simulink model "CPDemo"  (Simulink 7.8)
settings: Solver=ode1  StartTime=0  StopTime=250  FixedStep=1  RelTol=1e-3
libraries: DRRALibrary x105, simulink x10
settings Model: Creator=Administrator  LastModifiedBy=shuol
settings SolverCC: AlgebraicLoopSolver=LineSearch
settings OptimizationCC: BlockReduction=off  BooleanDataType=off  ConditionallyExecuteInputs=off

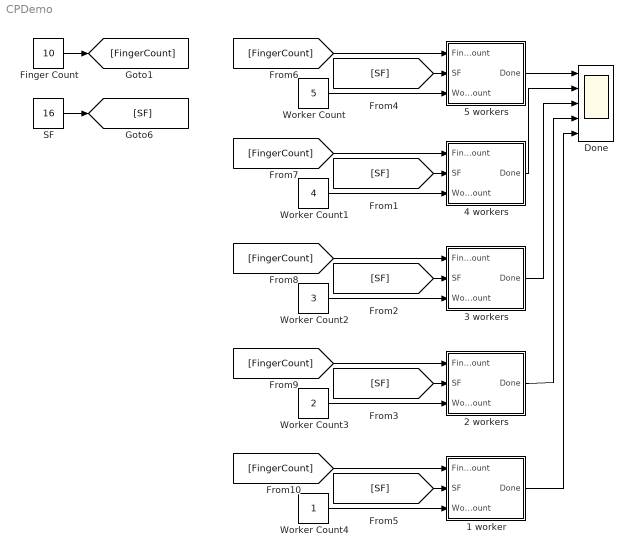
== system CPDemo ==
  1 worker : Subsystem
  2 workers : Subsystem
  3 workers : Subsystem
  4 workers : Subsystem
  5 workers : Subsystem
  Done : Scope  NumInputPorts=5
      settings: TickLabels=on  YMin=-1~-1~-1~-1~-1  YMax=2~2~2~2~2
  Finger Count : Constant  Value=10  SampleTime=1
  SF : Constant  Value=16  SampleTime=1
  Worker Count : Constant  Value=5  SampleTime=1
  Worker Count1 : Constant  Value=4  SampleTime=1
  Worker Count2 : Constant  Value=3  SampleTime=1
  Worker Count3 : Constant  Value=2  SampleTime=1
  Worker Count4 : Constant  SampleTime=1
  wires:
  [SF] -> 5 workers/2(SF)
  Worker Count/1 -> 5 workers/3(Worker Count)
  5 workers/1(Done) -> Done/1
  [SF] -> 4 workers/2(SF)
  Worker Count1/1 -> 4 workers/3(Worker Count)
  [SF] -> 3 workers/2(SF)
  Worker Count2/1 -> 3 workers/3(Worker Count)
  [SF] -> 2 workers/2(SF)
  Worker Count3/1 -> 2 workers/3(Worker Count)
  [SF] -> 1 worker/2(SF)
  Worker Count4/1 -> 1 worker/3(Worker Count)
  4 workers/1(Done) -> Done/2
  3 workers/1(Done) -> Done/3
  2 workers/1(Done) -> Done/4
  1 worker/1(Done) -> Done/5
  SF/1 -> [SF]
  Finger Count/1 -> [FingerCount]
  [FingerCount] -> 5 workers/1(Finger Count)
  [FingerCount] -> 1 worker/1(Finger Count)
  [FingerCount] -> 2 workers/1(Finger Count)
  [FingerCount] -> 3 workers/1(Finger Count)
  [FingerCount] -> 4 workers/1(Finger Count)

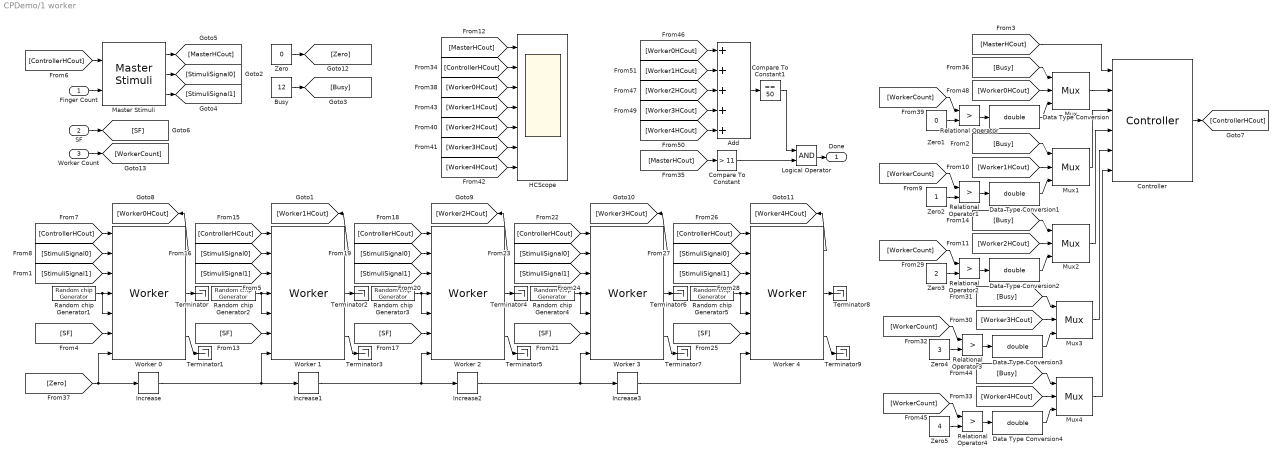
== system CPDemo/1 worker ==
  Finger Count : Inport
  SF : Inport  Port=2
  Worker Count : Inport  Port=3
  Add : Sum  Inputs=+++++  SampleTime=1
  Busy : Constant  Value=12  SampleTime=1
  Compare To Constant : simulink/Logic and Bit Operations/Compare To Constant  relop=>  const=11  OutDataTypeStr=uint8
  Compare To Constant1 : simulink/Logic and Bit Operations/Compare To Constant  relop===  const=50  OutDataTypeStr=uint8
  Controller : DRRALibrary/Function Library/Correlation Pool/Used Functions/Extended Functions/Controller
  Data Type Conversion{,1..4} (5 alike) : DataTypeConversion  OutDataTypeStr=double
  HCScope : Scope  NumInputPorts=7
      settings: TickLabels=on  YMin=-1~-1~-1~-1~-1~-1~-1  YMax=16~16~16~16~16~16~16
  Increase{,1..3} (4 alike) : DRRALibrary/Simulation Functions/Base Functions/Increase  SystemSampleTime=-1
  Logical Operator : Logic  AllPortsSameDT=off  OutDataTypeStr=boolean
  Master Stimuli : DRRALibrary/Function Library/Correlation Pool/Used Functions/Extended Functions/Master Stimuli
  Mux{,1..4} (5 alike) : DRRALibrary/Simulation Functions/Base Functions/Mux
  Random chip Generator{1..5} (5 alike) : DRRALibrary/Function Library/Correlation Pool/Used Functions/Extended Functions/Random chip Generator
  Relational Operator{,1..4} (5 alike) : RelationalOperator  Operator=>  OutDataTypeStr=boolean
  Terminator{,1..9} (10 alike) : Terminator
  Worker {0..4} (5 alike) : DRRALibrary/Function Library/Correlation Pool/Used Functions/Extended Functions/Worker 
  Zero : Constant  Value=0  SampleTime=1
  Zero1 : Constant  Value=0  SampleTime=1
  Zero2 : Constant  SampleTime=1
  Zero3 : Constant  Value=2  SampleTime=1
  Zero4 : Constant  Value=3  SampleTime=1
  Zero5 : Constant  Value=4  SampleTime=1
  Done : Outport
  wires:
  Data Type Conversion/1 -> Mux/3
  Relational Operator/1 -> Data Type Conversion/1
  Worker Count/1 -> [WorkerCount]
  [Zero] -> Worker 0/7, Increase/1
  Zero/1 -> [Zero]
  Busy/1 -> [Busy]
  Finger Count/1 -> Master Stimuli/2
  Worker 4/3 -> Terminator9/1
  Worker 4/2 -> Terminator8/1
  Worker 3/2 -> Terminator6/1
  Worker 3/3 -> Terminator7/1
  Worker 2/3 -> Terminator5/1
  Worker 2/2 -> Terminator4/1
  Worker 1/3 -> Terminator3/1
  Worker 1/2 -> Terminator2/1
  Worker 0/3 -> Terminator1/1
  Worker 0/2 -> Terminator/1
  SF/1 -> [SF]
  Master Stimuli/3 -> [StimuliSignal1]
  Worker 4/1 -> [Worker4HCout]
  Increase3/1 -> Worker 4/7
  [SF] -> Worker 4/6
  [StimuliSignal1] -> Worker 4/3
  Random chip Generator5/1 -> Worker 4/4, Worker 4/5
  [StimuliSignal0] -> Worker 4/2
  [ControllerHCout] -> Worker 4/1
  Worker 3/1 -> [Worker3HCout]
  Increase2/1 -> Worker 3/7, Increase3/1
  [SF] -> Worker 3/6
  [StimuliSignal1] -> Worker 3/3
  Random chip Generator4/1 -> Worker 3/5, Worker 3/4
  [StimuliSignal0] -> Worker 3/2
  [ControllerHCout] -> Worker 3/1
  Worker 2/1 -> [Worker2HCout]
  Increase1/1 -> Increase2/1, Worker 2/7
  [SF] -> Worker 2/6
  [StimuliSignal1] -> Worker 2/3
  Random chip Generator3/1 -> Worker 2/4, Worker 2/5
  [StimuliSignal0] -> Worker 2/2
  [ControllerHCout] -> Worker 2/1
  Worker 1/1 -> [Worker1HCout]
  Increase/1 -> Worker 1/7, Increase1/1
  [SF] -> Worker 1/6
  [StimuliSignal1] -> Worker 1/3
  Random chip Generator2/1 -> Worker 1/5, Worker 1/4
  [StimuliSignal0] -> Worker 1/2
  [ControllerHCout] -> Worker 1/1
  Worker 0/1 -> [Worker0HCout]
  [SF] -> Worker 0/6
  [StimuliSignal1] -> Worker 0/3
  [ControllerHCout] -> Master Stimuli/1
  Random chip Generator1/1 -> Worker 0/4, Worker 0/5
  [StimuliSignal0] -> Worker 0/2
  [ControllerHCout] -> Worker 0/1
  [MasterHCout] -> Controller/1
  Controller/1 -> [ControllerHCout]
  Master Stimuli/2 -> [StimuliSignal0]
  Master Stimuli/1 -> [MasterHCout]
  [MasterHCout] -> Compare To Constant/1
  [MasterHCout] -> HCScope/1
  [ControllerHCout] -> HCScope/2
  [Worker0HCout] -> Mux/2
  [WorkerCount] -> Relational Operator/1
  Zero1/1 -> Relational Operator/2
  [Worker4HCout] -> HCScope/7
  [Worker3HCout] -> HCScope/6
  [Worker2HCout] -> HCScope/5
  [Worker1HCout] -> HCScope/4
  [Worker0HCout] -> HCScope/3
  [Busy] -> Mux/1
  Data Type Conversion1/1 -> Mux1/3
  Relational Operator1/1 -> Data Type Conversion1/1
  [Worker1HCout] -> Mux1/2
  [WorkerCount] -> Relational Operator1/1
  Zero2/1 -> Relational Operator1/2
  [Busy] -> Mux1/1
  Data Type Conversion2/1 -> Mux2/3
  Relational Operator2/1 -> Data Type Conversion2/1
  [Worker2HCout] -> Mux2/2
  [WorkerCount] -> Relational Operator2/1
  Zero3/1 -> Relational Operator2/2
  [Busy] -> Mux2/1
  Data Type Conversion3/1 -> Mux3/3
  Relational Operator3/1 -> Data Type Conversion3/1
  [Worker3HCout] -> Mux3/2
  [WorkerCount] -> Relational Operator3/1
  Zero4/1 -> Relational Operator3/2
  [Busy] -> Mux3/1
  Data Type Conversion4/1 -> Mux4/3
  Relational Operator4/1 -> Data Type Conversion4/1
  [Worker4HCout] -> Mux4/2
  [WorkerCount] -> Relational Operator4/1
  Zero5/1 -> Relational Operator4/2
  [Busy] -> Mux4/1
  Mux/1 -> Controller/2
  Mux1/1 -> Controller/3
  Mux2/1 -> Controller/4
  Mux3/1 -> Controller/5
  Mux4/1 -> Controller/6
  [Worker0HCout] -> Add/1
  [Worker1HCout] -> Add/2
  [Worker2HCout] -> Add/3
  [Worker3HCout] -> Add/4
  [Worker4HCout] -> Add/5
  Add/1 -> Compare To Constant1/1
  Compare To Constant/1 -> Logical Operator/2
  Compare To Constant1/1 -> Logical Operator/1
  Logical Operator/1 -> Done/1

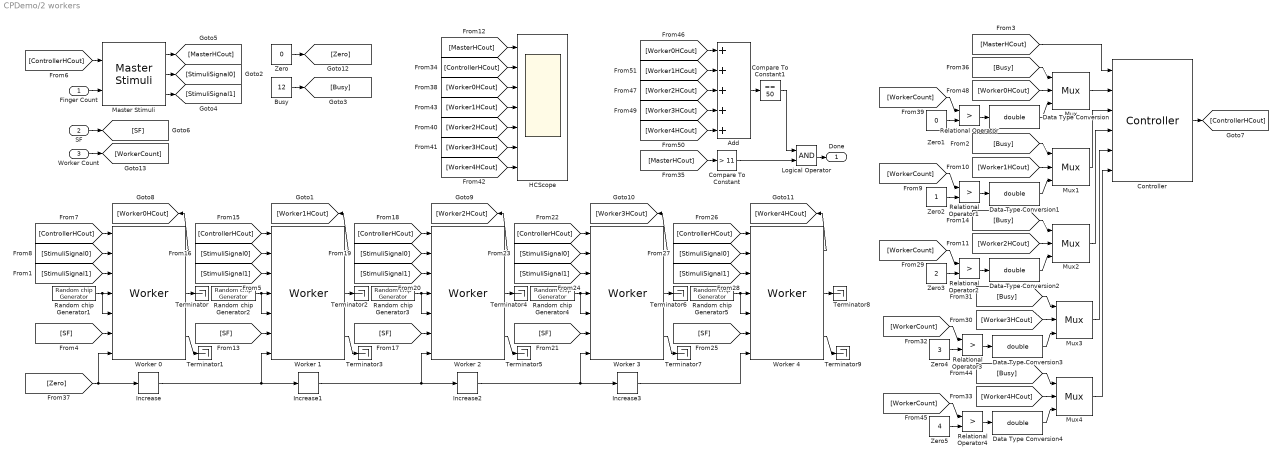
== system CPDemo/2 workers ==
  Finger Count : Inport
  SF : Inport  Port=2
  Worker Count : Inport  Port=3
  Add : Sum  Inputs=+++++  SampleTime=1
  Busy : Constant  Value=12  SampleTime=1
  Compare To Constant : simulink/Logic and Bit Operations/Compare To Constant  relop=>  const=11  OutDataTypeStr=uint8
  Compare To Constant1 : simulink/Logic and Bit Operations/Compare To Constant  relop===  const=50  OutDataTypeStr=uint8
  Controller : DRRALibrary/Function Library/Correlation Pool/Used Functions/Extended Functions/Controller
  Data Type Conversion{,1..4} (5 alike) : DataTypeConversion  OutDataTypeStr=double
  HCScope : Scope  NumInputPorts=7
      settings: TickLabels=on  YMin=-1~-1~-1~-1~-1~-1~-1  YMax=16~16~16~16~16~16~16
  Increase{,1..3} (4 alike) : DRRALibrary/Simulation Functions/Base Functions/Increase  SystemSampleTime=-1
  Logical Operator : Logic  AllPortsSameDT=off  OutDataTypeStr=boolean
  Master Stimuli : DRRALibrary/Function Library/Correlation Pool/Used Functions/Extended Functions/Master Stimuli
  Mux{,1..4} (5 alike) : DRRALibrary/Simulation Functions/Base Functions/Mux
  Random chip Generator{1..5} (5 alike) : DRRALibrary/Function Library/Correlation Pool/Used Functions/Extended Functions/Random chip Generator
  Relational Operator{,1..4} (5 alike) : RelationalOperator  Operator=>  OutDataTypeStr=boolean
  Terminator{,1..9} (10 alike) : Terminator
  Worker {0..4} (5 alike) : DRRALibrary/Function Library/Correlation Pool/Used Functions/Extended Functions/Worker 
  Zero : Constant  Value=0  SampleTime=1
  Zero1 : Constant  Value=0  SampleTime=1
  Zero2 : Constant  SampleTime=1
  Zero3 : Constant  Value=2  SampleTime=1
  Zero4 : Constant  Value=3  SampleTime=1
  Zero5 : Constant  Value=4  SampleTime=1
  Done : Outport
  wires:
  Logical Operator/1 -> Done/1
  Compare To Constant1/1 -> Logical Operator/1
  Compare To Constant/1 -> Logical Operator/2
  Add/1 -> Compare To Constant1/1
  [Worker4HCout] -> Add/5
  [Worker3HCout] -> Add/4
  [Worker2HCout] -> Add/3
  [Worker1HCout] -> Add/2
  [Worker0HCout] -> Add/1
  Mux4/1 -> Controller/6
  Mux3/1 -> Controller/5
  Mux2/1 -> Controller/4
  Mux1/1 -> Controller/3
  Mux/1 -> Controller/2
  [Busy] -> Mux4/1
  Zero5/1 -> Relational Operator4/2
  [WorkerCount] -> Relational Operator4/1
  [Worker4HCout] -> Mux4/2
  Relational Operator4/1 -> Data Type Conversion4/1
  Data Type Conversion4/1 -> Mux4/3
  [Busy] -> Mux3/1
  Zero4/1 -> Relational Operator3/2
  [WorkerCount] -> Relational Operator3/1
  [Worker3HCout] -> Mux3/2
  Relational Operator3/1 -> Data Type Conversion3/1
  Data Type Conversion3/1 -> Mux3/3
  [Busy] -> Mux2/1
  Zero3/1 -> Relational Operator2/2
  [WorkerCount] -> Relational Operator2/1
  [Worker2HCout] -> Mux2/2
  Relational Operator2/1 -> Data Type Conversion2/1
  Data Type Conversion2/1 -> Mux2/3
  [Busy] -> Mux1/1
  Zero2/1 -> Relational Operator1/2
  [WorkerCount] -> Relational Operator1/1
  [Worker1HCout] -> Mux1/2
  Relational Operator1/1 -> Data Type Conversion1/1
  Data Type Conversion1/1 -> Mux1/3
  [Busy] -> Mux/1
  [Worker0HCout] -> HCScope/3
  [Worker1HCout] -> HCScope/4
  [Worker2HCout] -> HCScope/5
  [Worker3HCout] -> HCScope/6
  [Worker4HCout] -> HCScope/7
  Zero1/1 -> Relational Operator/2
  [WorkerCount] -> Relational Operator/1
  [Worker0HCout] -> Mux/2
  [ControllerHCout] -> HCScope/2
  [MasterHCout] -> HCScope/1
  [MasterHCout] -> Compare To Constant/1
  Master Stimuli/1 -> [MasterHCout]
  Master Stimuli/2 -> [StimuliSignal0]
  Controller/1 -> [ControllerHCout]
  [MasterHCout] -> Controller/1
  [ControllerHCout] -> Worker 0/1
  [StimuliSignal0] -> Worker 0/2
  Random chip Generator1/1 -> Worker 0/5, Worker 0/4
  [ControllerHCout] -> Master Stimuli/1
  [StimuliSignal1] -> Worker 0/3
  [SF] -> Worker 0/6
  Worker 0/1 -> [Worker0HCout]
  [ControllerHCout] -> Worker 1/1
  [StimuliSignal0] -> Worker 1/2
  Random chip Generator2/1 -> Worker 1/4, Worker 1/5
  [StimuliSignal1] -> Worker 1/3
  [SF] -> Worker 1/6
  Increase/1 -> Increase1/1, Worker 1/7
  Worker 1/1 -> [Worker1HCout]
  [ControllerHCout] -> Worker 2/1
  [StimuliSignal0] -> Worker 2/2
  Random chip Generator3/1 -> Worker 2/5, Worker 2/4
  [StimuliSignal1] -> Worker 2/3
  [SF] -> Worker 2/6
  Increase1/1 -> Worker 2/7, Increase2/1
  Worker 2/1 -> [Worker2HCout]
  [ControllerHCout] -> Worker 3/1
  [StimuliSignal0] -> Worker 3/2
  Random chip Generator4/1 -> Worker 3/4, Worker 3/5
  [StimuliSignal1] -> Worker 3/3
  [SF] -> Worker 3/6
  Increase2/1 -> Increase3/1, Worker 3/7
  Worker 3/1 -> [Worker3HCout]
  [ControllerHCout] -> Worker 4/1
  [StimuliSignal0] -> Worker 4/2
  Random chip Generator5/1 -> Worker 4/5, Worker 4/4
  [StimuliSignal1] -> Worker 4/3
  [SF] -> Worker 4/6
  Increase3/1 -> Worker 4/7
  Worker 4/1 -> [Worker4HCout]
  Master Stimuli/3 -> [StimuliSignal1]
  SF/1 -> [SF]
  Worker 0/2 -> Terminator/1
  Worker 0/3 -> Terminator1/1
  Worker 1/2 -> Terminator2/1
  Worker 1/3 -> Terminator3/1
  Worker 2/2 -> Terminator4/1
  Worker 2/3 -> Terminator5/1
  Worker 3/3 -> Terminator7/1
  Worker 3/2 -> Terminator6/1
  Worker 4/2 -> Terminator8/1
  Worker 4/3 -> Terminator9/1
  Finger Count/1 -> Master Stimuli/2
  Busy/1 -> [Busy]
  Zero/1 -> [Zero]
  [Zero] -> Increase/1, Worker 0/7
  Worker Count/1 -> [WorkerCount]
  Relational Operator/1 -> Data Type Conversion/1
  Data Type Conversion/1 -> Mux/3

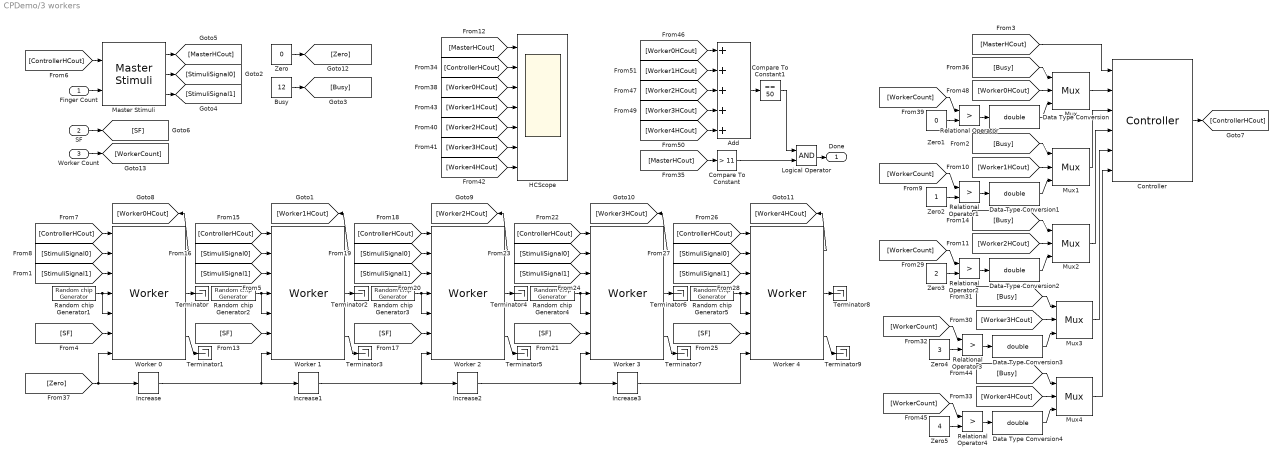
== system CPDemo/3 workers ==
  Finger Count : Inport
  SF : Inport  Port=2
  Worker Count : Inport  Port=3
  Add : Sum  Inputs=+++++  SampleTime=1
  Busy : Constant  Value=12  SampleTime=1
  Compare To Constant : simulink/Logic and Bit Operations/Compare To Constant  relop=>  const=11  OutDataTypeStr=uint8
  Compare To Constant1 : simulink/Logic and Bit Operations/Compare To Constant  relop===  const=50  OutDataTypeStr=uint8
  Controller : DRRALibrary/Function Library/Correlation Pool/Used Functions/Extended Functions/Controller
  Data Type Conversion{,1..4} (5 alike) : DataTypeConversion  OutDataTypeStr=double
  HCScope : Scope  NumInputPorts=7
      settings: TickLabels=on  YMin=-1~-1~-1~-1~-1~-1~-1  YMax=16~16~16~16~16~16~16
  Increase{,1..3} (4 alike) : DRRALibrary/Simulation Functions/Base Functions/Increase  SystemSampleTime=-1
  Logical Operator : Logic  AllPortsSameDT=off  OutDataTypeStr=boolean
  Master Stimuli : DRRALibrary/Function Library/Correlation Pool/Used Functions/Extended Functions/Master Stimuli
  Mux{,1..4} (5 alike) : DRRALibrary/Simulation Functions/Base Functions/Mux
  Random chip Generator{1..5} (5 alike) : DRRALibrary/Function Library/Correlation Pool/Used Functions/Extended Functions/Random chip Generator
  Relational Operator{,1..4} (5 alike) : RelationalOperator  Operator=>  OutDataTypeStr=boolean
  Terminator{,1..9} (10 alike) : Terminator
  Worker {0..4} (5 alike) : DRRALibrary/Function Library/Correlation Pool/Used Functions/Extended Functions/Worker 
  Zero : Constant  Value=0  SampleTime=1
  Zero1 : Constant  Value=0  SampleTime=1
  Zero2 : Constant  SampleTime=1
  Zero3 : Constant  Value=2  SampleTime=1
  Zero4 : Constant  Value=3  SampleTime=1
  Zero5 : Constant  Value=4  SampleTime=1
  Done : Outport
  wires:
  Data Type Conversion/1 -> Mux/3
  Relational Operator/1 -> Data Type Conversion/1
  Worker Count/1 -> [WorkerCount]
  [Zero] -> Worker 0/7, Increase/1
  Zero/1 -> [Zero]
  Busy/1 -> [Busy]
  Finger Count/1 -> Master Stimuli/2
  Worker 4/3 -> Terminator9/1
  Worker 4/2 -> Terminator8/1
  Worker 3/2 -> Terminator6/1
  Worker 3/3 -> Terminator7/1
  Worker 2/3 -> Terminator5/1
  Worker 2/2 -> Terminator4/1
  Worker 1/3 -> Terminator3/1
  Worker 1/2 -> Terminator2/1
  Worker 0/3 -> Terminator1/1
  Worker 0/2 -> Terminator/1
  SF/1 -> [SF]
  Master Stimuli/3 -> [StimuliSignal1]
  Worker 4/1 -> [Worker4HCout]
  Increase3/1 -> Worker 4/7
  [SF] -> Worker 4/6
  [StimuliSignal1] -> Worker 4/3
  Random chip Generator5/1 -> Worker 4/4, Worker 4/5
  [StimuliSignal0] -> Worker 4/2
  [ControllerHCout] -> Worker 4/1
  Worker 3/1 -> [Worker3HCout]
  Increase2/1 -> Worker 3/7, Increase3/1
  [SF] -> Worker 3/6
  [StimuliSignal1] -> Worker 3/3
  Random chip Generator4/1 -> Worker 3/5, Worker 3/4
  [StimuliSignal0] -> Worker 3/2
  [ControllerHCout] -> Worker 3/1
  Worker 2/1 -> [Worker2HCout]
  Increase1/1 -> Increase2/1, Worker 2/7
  [SF] -> Worker 2/6
  [StimuliSignal1] -> Worker 2/3
  Random chip Generator3/1 -> Worker 2/4, Worker 2/5
  [StimuliSignal0] -> Worker 2/2
  [ControllerHCout] -> Worker 2/1
  Worker 1/1 -> [Worker1HCout]
  Increase/1 -> Worker 1/7, Increase1/1
  [SF] -> Worker 1/6
  [StimuliSignal1] -> Worker 1/3
  Random chip Generator2/1 -> Worker 1/5, Worker 1/4
  [StimuliSignal0] -> Worker 1/2
  [ControllerHCout] -> Worker 1/1
  Worker 0/1 -> [Worker0HCout]
  [SF] -> Worker 0/6
  [StimuliSignal1] -> Worker 0/3
  [ControllerHCout] -> Master Stimuli/1
  Random chip Generator1/1 -> Worker 0/4, Worker 0/5
  [StimuliSignal0] -> Worker 0/2
  [ControllerHCout] -> Worker 0/1
  [MasterHCout] -> Controller/1
  Controller/1 -> [ControllerHCout]
  Master Stimuli/2 -> [StimuliSignal0]
  Master Stimuli/1 -> [MasterHCout]
  [MasterHCout] -> Compare To Constant/1
  [MasterHCout] -> HCScope/1
  [ControllerHCout] -> HCScope/2
  [Worker0HCout] -> Mux/2
  [WorkerCount] -> Relational Operator/1
  Zero1/1 -> Relational Operator/2
  [Worker4HCout] -> HCScope/7
  [Worker3HCout] -> HCScope/6
  [Worker2HCout] -> HCScope/5
  [Worker1HCout] -> HCScope/4
  [Worker0HCout] -> HCScope/3
  [Busy] -> Mux/1
  Data Type Conversion1/1 -> Mux1/3
  Relational Operator1/1 -> Data Type Conversion1/1
  [Worker1HCout] -> Mux1/2
  [WorkerCount] -> Relational Operator1/1
  Zero2/1 -> Relational Operator1/2
  [Busy] -> Mux1/1
  Data Type Conversion2/1 -> Mux2/3
  Relational Operator2/1 -> Data Type Conversion2/1
  [Worker2HCout] -> Mux2/2
  [WorkerCount] -> Relational Operator2/1
  Zero3/1 -> Relational Operator2/2
  [Busy] -> Mux2/1
  Data Type Conversion3/1 -> Mux3/3
  Relational Operator3/1 -> Data Type Conversion3/1
  [Worker3HCout] -> Mux3/2
  [WorkerCount] -> Relational Operator3/1
  Zero4/1 -> Relational Operator3/2
  [Busy] -> Mux3/1
  Data Type Conversion4/1 -> Mux4/3
  Relational Operator4/1 -> Data Type Conversion4/1
  [Worker4HCout] -> Mux4/2
  [WorkerCount] -> Relational Operator4/1
  Zero5/1 -> Relational Operator4/2
  [Busy] -> Mux4/1
  Mux/1 -> Controller/2
  Mux1/1 -> Controller/3
  Mux2/1 -> Controller/4
  Mux3/1 -> Controller/5
  Mux4/1 -> Controller/6
  [Worker0HCout] -> Add/1
  [Worker1HCout] -> Add/2
  [Worker2HCout] -> Add/3
  [Worker3HCout] -> Add/4
  [Worker4HCout] -> Add/5
  Add/1 -> Compare To Constant1/1
  Compare To Constant/1 -> Logical Operator/2
  Compare To Constant1/1 -> Logical Operator/1
  Logical Operator/1 -> Done/1

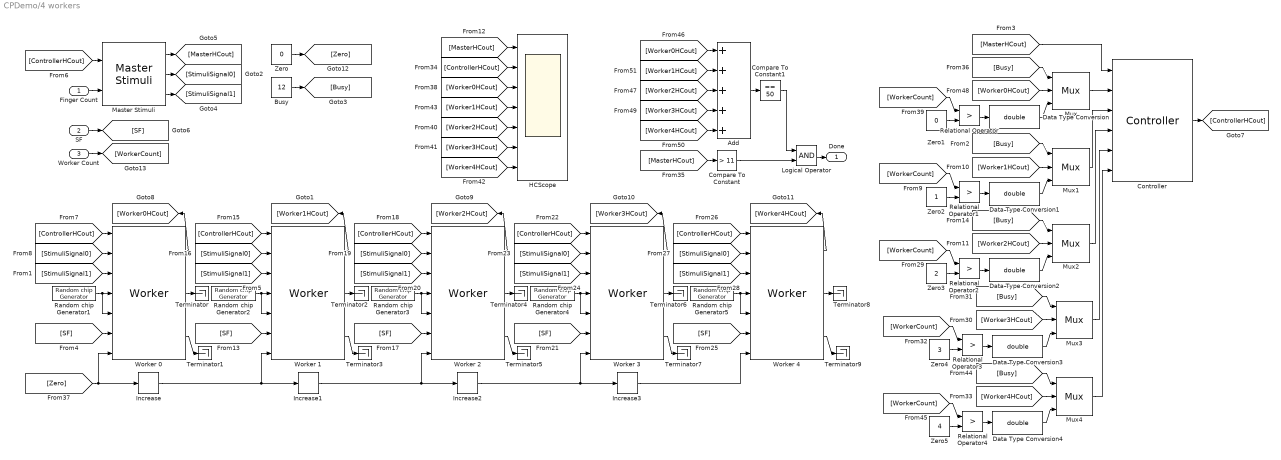
== system CPDemo/4 workers ==
  Finger Count : Inport
  SF : Inport  Port=2
  Worker Count : Inport  Port=3
  Add : Sum  Inputs=+++++  SampleTime=1
  Busy : Constant  Value=12  SampleTime=1
  Compare To Constant : simulink/Logic and Bit Operations/Compare To Constant  relop=>  const=11  OutDataTypeStr=uint8
  Compare To Constant1 : simulink/Logic and Bit Operations/Compare To Constant  relop===  const=50  OutDataTypeStr=uint8
  Controller : DRRALibrary/Function Library/Correlation Pool/Used Functions/Extended Functions/Controller
  Data Type Conversion{,1..4} (5 alike) : DataTypeConversion  OutDataTypeStr=double
  HCScope : Scope  NumInputPorts=7
      settings: TickLabels=on  YMin=-1~-1~-1~-1~-1~-1~-1  YMax=16~16~16~16~16~16~16
  Increase{,1..3} (4 alike) : DRRALibrary/Simulation Functions/Base Functions/Increase  SystemSampleTime=-1
  Logical Operator : Logic  AllPortsSameDT=off  OutDataTypeStr=boolean
  Master Stimuli : DRRALibrary/Function Library/Correlation Pool/Used Functions/Extended Functions/Master Stimuli
  Mux{,1..4} (5 alike) : DRRALibrary/Simulation Functions/Base Functions/Mux
  Random chip Generator{1..5} (5 alike) : DRRALibrary/Function Library/Correlation Pool/Used Functions/Extended Functions/Random chip Generator
  Relational Operator{,1..4} (5 alike) : RelationalOperator  Operator=>  OutDataTypeStr=boolean
  Terminator{,1..9} (10 alike) : Terminator
  Worker {0..4} (5 alike) : DRRALibrary/Function Library/Correlation Pool/Used Functions/Extended Functions/Worker 
  Zero : Constant  Value=0  SampleTime=1
  Zero1 : Constant  Value=0  SampleTime=1
  Zero2 : Constant  SampleTime=1
  Zero3 : Constant  Value=2  SampleTime=1
  Zero4 : Constant  Value=3  SampleTime=1
  Zero5 : Constant  Value=4  SampleTime=1
  Done : Outport
  wires:
  Logical Operator/1 -> Done/1
  Compare To Constant1/1 -> Logical Operator/1
  Compare To Constant/1 -> Logical Operator/2
  Add/1 -> Compare To Constant1/1
  [Worker4HCout] -> Add/5
  [Worker3HCout] -> Add/4
  [Worker2HCout] -> Add/3
  [Worker1HCout] -> Add/2
  [Worker0HCout] -> Add/1
  Mux4/1 -> Controller/6
  Mux3/1 -> Controller/5
  Mux2/1 -> Controller/4
  Mux1/1 -> Controller/3
  Mux/1 -> Controller/2
  [Busy] -> Mux4/1
  Zero5/1 -> Relational Operator4/2
  [WorkerCount] -> Relational Operator4/1
  [Worker4HCout] -> Mux4/2
  Relational Operator4/1 -> Data Type Conversion4/1
  Data Type Conversion4/1 -> Mux4/3
  [Busy] -> Mux3/1
  Zero4/1 -> Relational Operator3/2
  [WorkerCount] -> Relational Operator3/1
  [Worker3HCout] -> Mux3/2
  Relational Operator3/1 -> Data Type Conversion3/1
  Data Type Conversion3/1 -> Mux3/3
  [Busy] -> Mux2/1
  Zero3/1 -> Relational Operator2/2
  [WorkerCount] -> Relational Operator2/1
  [Worker2HCout] -> Mux2/2
  Relational Operator2/1 -> Data Type Conversion2/1
  Data Type Conversion2/1 -> Mux2/3
  [Busy] -> Mux1/1
  Zero2/1 -> Relational Operator1/2
  [WorkerCount] -> Relational Operator1/1
  [Worker1HCout] -> Mux1/2
  Relational Operator1/1 -> Data Type Conversion1/1
  Data Type Conversion1/1 -> Mux1/3
  [Busy] -> Mux/1
  [Worker0HCout] -> HCScope/3
  [Worker1HCout] -> HCScope/4
  [Worker2HCout] -> HCScope/5
  [Worker3HCout] -> HCScope/6
  [Worker4HCout] -> HCScope/7
  Zero1/1 -> Relational Operator/2
  [WorkerCount] -> Relational Operator/1
  [Worker0HCout] -> Mux/2
  [ControllerHCout] -> HCScope/2
  [MasterHCout] -> HCScope/1
  [MasterHCout] -> Compare To Constant/1
  Master Stimuli/1 -> [MasterHCout]
  Master Stimuli/2 -> [StimuliSignal0]
  Controller/1 -> [ControllerHCout]
  [MasterHCout] -> Controller/1
  [ControllerHCout] -> Worker 0/1
  [StimuliSignal0] -> Worker 0/2
  Random chip Generator1/1 -> Worker 0/5, Worker 0/4
  [ControllerHCout] -> Master Stimuli/1
  [StimuliSignal1] -> Worker 0/3
  [SF] -> Worker 0/6
  Worker 0/1 -> [Worker0HCout]
  [ControllerHCout] -> Worker 1/1
  [StimuliSignal0] -> Worker 1/2
  Random chip Generator2/1 -> Worker 1/4, Worker 1/5
  [StimuliSignal1] -> Worker 1/3
  [SF] -> Worker 1/6
  Increase/1 -> Increase1/1, Worker 1/7
  Worker 1/1 -> [Worker1HCout]
  [ControllerHCout] -> Worker 2/1
  [StimuliSignal0] -> Worker 2/2
  Random chip Generator3/1 -> Worker 2/5, Worker 2/4
  [StimuliSignal1] -> Worker 2/3
  [SF] -> Worker 2/6
  Increase1/1 -> Worker 2/7, Increase2/1
  Worker 2/1 -> [Worker2HCout]
  [ControllerHCout] -> Worker 3/1
  [StimuliSignal0] -> Worker 3/2
  Random chip Generator4/1 -> Worker 3/4, Worker 3/5
  [StimuliSignal1] -> Worker 3/3
  [SF] -> Worker 3/6
  Increase2/1 -> Increase3/1, Worker 3/7
  Worker 3/1 -> [Worker3HCout]
  [ControllerHCout] -> Worker 4/1
  [StimuliSignal0] -> Worker 4/2
  Random chip Generator5/1 -> Worker 4/5, Worker 4/4
  [StimuliSignal1] -> Worker 4/3
  [SF] -> Worker 4/6
  Increase3/1 -> Worker 4/7
  Worker 4/1 -> [Worker4HCout]
  Master Stimuli/3 -> [StimuliSignal1]
  SF/1 -> [SF]
  Worker 0/2 -> Terminator/1
  Worker 0/3 -> Terminator1/1
  Worker 1/2 -> Terminator2/1
  Worker 1/3 -> Terminator3/1
  Worker 2/2 -> Terminator4/1
  Worker 2/3 -> Terminator5/1
  Worker 3/3 -> Terminator7/1
  Worker 3/2 -> Terminator6/1
  Worker 4/2 -> Terminator8/1
  Worker 4/3 -> Terminator9/1
  Finger Count/1 -> Master Stimuli/2
  Busy/1 -> [Busy]
  Zero/1 -> [Zero]
  [Zero] -> Increase/1, Worker 0/7
  Worker Count/1 -> [WorkerCount]
  Relational Operator/1 -> Data Type Conversion/1
  Data Type Conversion/1 -> Mux/3

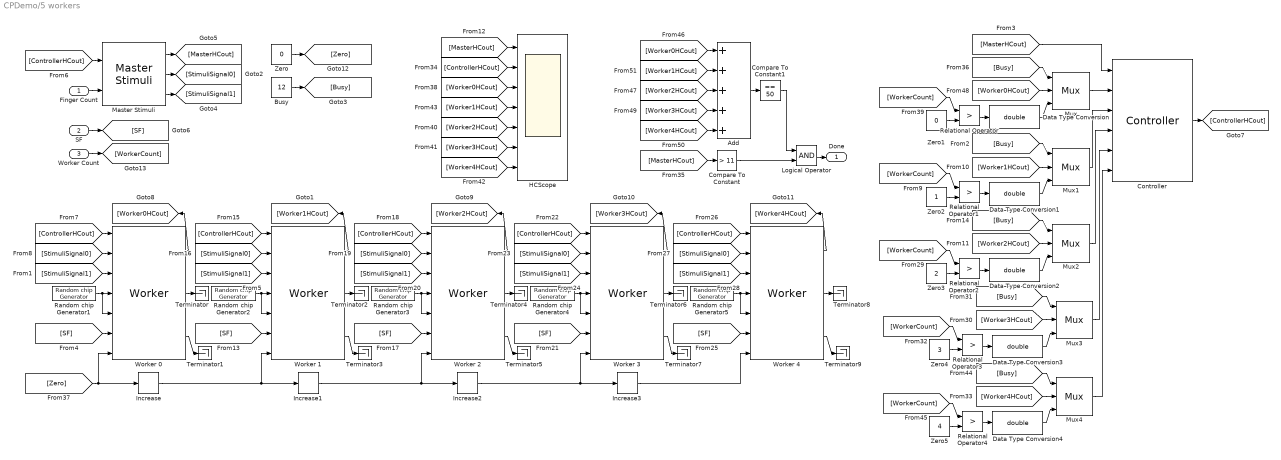
== system CPDemo/5 workers ==
  Finger Count : Inport
  SF : Inport  Port=2
  Worker Count : Inport  Port=3
  Add : Sum  Inputs=+++++  SampleTime=1
  Busy : Constant  Value=12  SampleTime=1
  Compare To Constant : simulink/Logic and Bit Operations/Compare To Constant  relop=>  const=11  OutDataTypeStr=uint8
  Compare To Constant1 : simulink/Logic and Bit Operations/Compare To Constant  relop===  const=50  OutDataTypeStr=uint8
  Controller : DRRALibrary/Function Library/Correlation Pool/Used Functions/Extended Functions/Controller
  Data Type Conversion{,1..4} (5 alike) : DataTypeConversion  OutDataTypeStr=double
  HCScope : Scope  NumInputPorts=7
      settings: TickLabels=on  YMin=-1~-1~-1~-1~-1~-1~-1  YMax=16~16~16~16~16~16~16
  Increase{,1..3} (4 alike) : DRRALibrary/Simulation Functions/Base Functions/Increase  SystemSampleTime=-1
  Logical Operator : Logic  AllPortsSameDT=off  OutDataTypeStr=boolean
  Master Stimuli : DRRALibrary/Function Library/Correlation Pool/Used Functions/Extended Functions/Master Stimuli
  Mux{,1..4} (5 alike) : DRRALibrary/Simulation Functions/Base Functions/Mux
  Random chip Generator{1..5} (5 alike) : DRRALibrary/Function Library/Correlation Pool/Used Functions/Extended Functions/Random chip Generator
  Relational Operator{,1..4} (5 alike) : RelationalOperator  Operator=>  OutDataTypeStr=boolean
  Terminator{,1..9} (10 alike) : Terminator
  Worker {0..4} (5 alike) : DRRALibrary/Function Library/Correlation Pool/Used Functions/Extended Functions/Worker 
  Zero : Constant  Value=0  SampleTime=1
  Zero1 : Constant  Value=0  SampleTime=1
  Zero2 : Constant  SampleTime=1
  Zero3 : Constant  Value=2  SampleTime=1
  Zero4 : Constant  Value=3  SampleTime=1
  Zero5 : Constant  Value=4  SampleTime=1
  Done : Outport
  wires:
  Data Type Conversion/1 -> Mux/3
  Relational Operator/1 -> Data Type Conversion/1
  Worker Count/1 -> [WorkerCount]
  [Zero] -> Worker 0/7, Increase/1
  Zero/1 -> [Zero]
  Busy/1 -> [Busy]
  Finger Count/1 -> Master Stimuli/2
  Worker 4/3 -> Terminator9/1
  Worker 4/2 -> Terminator8/1
  Worker 3/2 -> Terminator6/1
  Worker 3/3 -> Terminator7/1
  Worker 2/3 -> Terminator5/1
  Worker 2/2 -> Terminator4/1
  Worker 1/3 -> Terminator3/1
  Worker 1/2 -> Terminator2/1
  Worker 0/3 -> Terminator1/1
  Worker 0/2 -> Terminator/1
  SF/1 -> [SF]
  Master Stimuli/3 -> [StimuliSignal1]
  Worker 4/1 -> [Worker4HCout]
  Increase3/1 -> Worker 4/7
  [SF] -> Worker 4/6
  [StimuliSignal1] -> Worker 4/3
  Random chip Generator5/1 -> Worker 4/4, Worker 4/5
  [StimuliSignal0] -> Worker 4/2
  [ControllerHCout] -> Worker 4/1
  Worker 3/1 -> [Worker3HCout]
  Increase2/1 -> Worker 3/7, Increase3/1
  [SF] -> Worker 3/6
  [StimuliSignal1] -> Worker 3/3
  Random chip Generator4/1 -> Worker 3/5, Worker 3/4
  [StimuliSignal0] -> Worker 3/2
  [ControllerHCout] -> Worker 3/1
  Worker 2/1 -> [Worker2HCout]
  Increase1/1 -> Increase2/1, Worker 2/7
  [SF] -> Worker 2/6
  [StimuliSignal1] -> Worker 2/3
  Random chip Generator3/1 -> Worker 2/4, Worker 2/5
  [StimuliSignal0] -> Worker 2/2
  [ControllerHCout] -> Worker 2/1
  Worker 1/1 -> [Worker1HCout]
  Increase/1 -> Worker 1/7, Increase1/1
  [SF] -> Worker 1/6
  [StimuliSignal1] -> Worker 1/3
  Random chip Generator2/1 -> Worker 1/5, Worker 1/4
  [StimuliSignal0] -> Worker 1/2
  [ControllerHCout] -> Worker 1/1
  Worker 0/1 -> [Worker0HCout]
  [SF] -> Worker 0/6
  [StimuliSignal1] -> Worker 0/3
  [ControllerHCout] -> Master Stimuli/1
  Random chip Generator1/1 -> Worker 0/4, Worker 0/5
  [StimuliSignal0] -> Worker 0/2
  [ControllerHCout] -> Worker 0/1
  [MasterHCout] -> Controller/1
  Controller/1 -> [ControllerHCout]
  Master Stimuli/2 -> [StimuliSignal0]
  Master Stimuli/1 -> [MasterHCout]
  [MasterHCout] -> Compare To Constant/1
  [MasterHCout] -> HCScope/1
  [ControllerHCout] -> HCScope/2
  [Worker0HCout] -> Mux/2
  [WorkerCount] -> Relational Operator/1
  Zero1/1 -> Relational Operator/2
  [Worker4HCout] -> HCScope/7
  [Worker3HCout] -> HCScope/6
  [Worker2HCout] -> HCScope/5
  [Worker1HCout] -> HCScope/4
  [Worker0HCout] -> HCScope/3
  [Busy] -> Mux/1
  Data Type Conversion1/1 -> Mux1/3
  Relational Operator1/1 -> Data Type Conversion1/1
  [Worker1HCout] -> Mux1/2
  [WorkerCount] -> Relational Operator1/1
  Zero2/1 -> Relational Operator1/2
  [Busy] -> Mux1/1
  Data Type Conversion2/1 -> Mux2/3
  Relational Operator2/1 -> Data Type Conversion2/1
  [Worker2HCout] -> Mux2/2
  [WorkerCount] -> Relational Operator2/1
  Zero3/1 -> Relational Operator2/2
  [Busy] -> Mux2/1
  Data Type Conversion3/1 -> Mux3/3
  Relational Operator3/1 -> Data Type Conversion3/1
  [Worker3HCout] -> Mux3/2
  [WorkerCount] -> Relational Operator3/1
  Zero4/1 -> Relational Operator3/2
  [Busy] -> Mux3/1
  Data Type Conversion4/1 -> Mux4/3
  Relational Operator4/1 -> Data Type Conversion4/1
  [Worker4HCout] -> Mux4/2
  [WorkerCount] -> Relational Operator4/1
  Zero5/1 -> Relational Operator4/2
  [Busy] -> Mux4/1
  Mux/1 -> Controller/2
  Mux1/1 -> Controller/3
  Mux2/1 -> Controller/4
  Mux3/1 -> Controller/5
  Mux4/1 -> Controller/6
  [Worker0HCout] -> Add/1
  [Worker1HCout] -> Add/2
  [Worker2HCout] -> Add/3
  [Worker3HCout] -> Add/4
  [Worker4HCout] -> Add/5
  Add/1 -> Compare To Constant1/1
  Compare To Constant/1 -> Logical Operator/2
  Compare To Constant1/1 -> Logical Operator/1
  Logical Operator/1 -> Done/1
